simulink model "Simulacion_2"  (R2021b)
settings: Solver=VariableStepAuto  StartTime=0.0  StopTime=1/60  MaxStep=0.0001  MinStep=0.00001  RelTol=1e-3
libraries: spsSeriesRLCBranchLib x6, spsACVoltageSourceLib x3, spsCurrentMeasurementLib x3, spsPowerLib x3, spsVoltageMeasurementLib x3, spsNeutralLib x1, spspowerguiLib x1
settings Model: Creator=Roberto  LastModifiedBy=Roberto

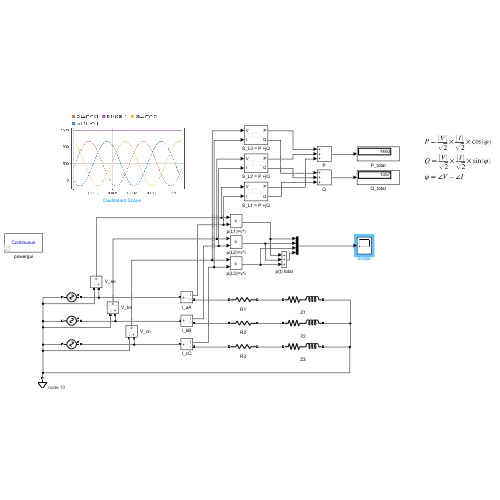
[thumbnail: Simulink's stored preview of the top-level diagram]
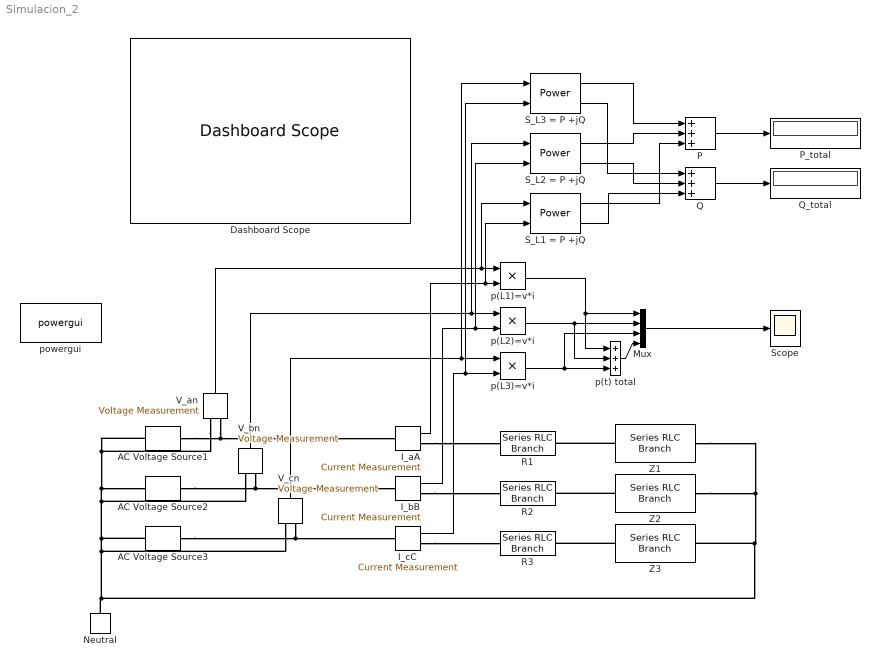
== system Simulacion_2 ==
  AC Voltage Source1 : spsACVoltageSourceLib/AC Voltage Source  Amplitude=100  Phase=0  Frequency=60  SampleTime=0  Measurements=None  BusType=swing  Pref=10e3  Qref=0  Qmin=-inf  Qmax=+inf
  AC Voltage Source2 : spsACVoltageSourceLib/AC Voltage Source  Amplitude=100  Phase=240  Frequency=60  SampleTime=0  Measurements=None  BusType=swing  Pref=10e3  Qref=0  Qmin=-inf  Qmax=+inf
  AC Voltage Source3 : spsACVoltageSourceLib/AC Voltage Source  Amplitude=100  Phase=120  Frequency=60  SampleTime=0  Measurements=None  BusType=swing  Pref=10e3  Qref=0  Qmin=-inf  Qmax=+inf
  Dashboard Scope : DashboardScope
  I_aA : spsCurrentMeasurementLib/Current Measurement  PhasorSimulation=off  OutputType=Complex  PSBequivalent=0
  I_bB : spsCurrentMeasurementLib/Current Measurement  PhasorSimulation=off  OutputType=Complex  PSBequivalent=0
  I_cC : spsCurrentMeasurementLib/Current Measurement  PhasorSimulation=off  OutputType=Complex  PSBequivalent=0
  Mux : Mux
  Neutral : spsNeutralLib/Neutral  LConnTagsString=a  NodeNumber=10
      settings: AttributesFormatString=node %<NodeNumber>  SourceProductBaseCode=PS
  P : Sum  Inputs=+++
  P_total : Display
  Q : Sum  Inputs=+++
  Q_total : Display
  R1 : spsSeriesRLCBranchLib/Series RLC Branch  LConnTagsString=__new0  RConnTagsString=__new0  BranchType=R  Resistance=0.5  Inductance=1e-3  SetiL0=off  InitialCurrent=0  Capacitance=1e-6  Setx0=off  InitialVoltage=0  Measurements=None
  R2 : spsSeriesRLCBranchLib/Series RLC Branch  LConnTagsString=__new0  RConnTagsString=__new0  BranchType=R  Resistance=0.5  Inductance=1e-3  SetiL0=off  InitialCurrent=0  Capacitance=1e-6  Setx0=off  InitialVoltage=0  Measurements=None
  R3 : spsSeriesRLCBranchLib/Series RLC Branch  LConnTagsString=__new0  RConnTagsString=__new0  BranchType=R  Resistance=0.5  Inductance=1e-3  SetiL0=off  InitialCurrent=0  Capacitance=1e-6  Setx0=off  InitialVoltage=0  Measurements=None
  S_L1 = P +jQ : spsPowerLib/Power  Freq=60  Vinit=[1, 0]  Iinit=[1, 0]  Ts=0
      settings: SourceProductBaseCode=PS
  S_L2 = P +jQ : spsPowerLib/Power  Freq=60  Vinit=[1, 0]  Iinit=[1, 0]  Ts=0
      settings: SourceProductBaseCode=PS
  S_L3 = P +jQ : spsPowerLib/Power  Freq=60  Vinit=[1, 0]  Iinit=[1, 0]  Ts=0
      settings: SourceProductBaseCode=PS
  Scope : Scope
  V_an : spsVoltageMeasurementLib/Voltage Measurement  PhasorSimulation=off  OutputType=Complex  PSBequivalent=0
  V_bn : spsVoltageMeasurementLib/Voltage Measurement  PhasorSimulation=off  OutputType=Complex  PSBequivalent=0
  V_cn : spsVoltageMeasurementLib/Voltage Measurement  PhasorSimulation=off  OutputType=Complex  PSBequivalent=0
  Z1 : spsSeriesRLCBranchLib/Series RLC Branch  LConnTagsString=__new0  RConnTagsString=__new0  BranchType=RL  Resistance=5  Inductance=5/(2*pi*60)  SetiL0=off  InitialCurrent=0  Capacitance=1e-6  Setx0=off  InitialVoltage=0  Measurements=None
  Z2 : spsSeriesRLCBranchLib/Series RLC Branch  LConnTagsString=__new0  RConnTagsString=__new0  BranchType=RL  Resistance=5  Inductance=5/(2*pi*60)  SetiL0=off  InitialCurrent=0  Capacitance=1e-6  Setx0=off  InitialVoltage=0  Measurements=None
  Z3 : spsSeriesRLCBranchLib/Series RLC Branch  LConnTagsString=__new0  RConnTagsString=__new0  BranchType=RL  Resistance=5  Inductance=5/(2*pi*60)  SetiL0=off  InitialCurrent=0  Capacitance=1e-6  Setx0=off  InitialVoltage=0  Measurements=None
  p(L1)=v*i : Product
  p(L2)=v*i : Product
  p(L3)=v*i : Product
  p(t) total : Sum  Inputs=+++
  powergui : spspowerguiLib/powergui  Priority=1  SimulationMode=Continuous  SampleTime=50e-6  frequency=60  Iterations=50  frequencyindice=60  Pbase=100e6  ErrMax=1e-4  UnitsV=kV  UnitsW=MW  buscounter=0  FunctionMessages=off  echomessages=off  EnableUseOfTLC=off  CurrentSourceSwitches=off  DisableSnubberDevices=off  DisableRonSwitches=off  DisableVfSwitches=off  DisplayEquations=off  AutomaticDiscreteSolvers=off  SolverType=Tustin/Backward Euler (TBE)  Interpol=off  ExternalGateDelay=off  methode=off  Ts=100  x0status=blocks  SPID=on  SwTol=0  HookPort=off  NonlinearTolerance=1e-4  nMaxIteration=100  ContinueOnMaxIteration=off  RestoreLinks=warning  ResistiveCurrentMeasurement=off  Frange=[0:2:500]  Ylog=off  Xlog=on  ShowGrid=off  save=off  variable=ZData  structure=0  ZoomFFT=off  StartTime=0.0  cycles=1  DisplayStyle=1  fundamental=60  FreqAxis=off  MaxFrequency=1000  frequencyindicesteady=1  RmsSteady=1  display=off
  wires:
  V_cn/1 -> S_L3 = P +jQ/1, p(L3)=v*i/1
  V_bn/1 -> S_L2 = P +jQ/1, p(L2)=v*i/1
  V_an/1 -> S_L1 = P +jQ/1, p(L1)=v*i/1
  I_aA/1 -> S_L1 = P +jQ/2, p(L1)=v*i/2
  I_cC/1 -> S_L3 = P +jQ/2, p(L3)=v*i/2
  p(L2)=v*i/1 -> p(t) total/2, Mux/2
  p(L3)=v*i/1 -> Mux/3, p(t) total/3
  p(t) total/1 -> Mux/4
  p(L1)=v*i/1 -> Mux/1, p(t) total/1
  I_bB/1 -> S_L2 = P +jQ/2, p(L2)=v*i/2
  S_L3 = P +jQ/1 -> P/1
  S_L2 = P +jQ/1 -> P/2
  S_L1 = P +jQ/1 -> P/3
  S_L3 = P +jQ/2 -> Q/1
  S_L2 = P +jQ/2 -> Q/2
  S_L1 = P +jQ/2 -> Q/3
  Q/1 -> Q_total/1
  P/1 -> P_total/1
  Mux/1 -> Scope/1
  connections:
  I_cC/RConn1 -- R3/LConn1
  I_bB/RConn1 -- R2/LConn1
  I_aA/RConn1 -- R1/LConn1
  AC Voltage Source1/RConn1 -- V_an/LConn1 -- I_aA/LConn1
  AC Voltage Source2/RConn1 -- V_bn/LConn1 -- I_bB/LConn1
  AC Voltage Source3/RConn1 -- V_cn/LConn1 -- I_cC/LConn1
  Z1/LConn1 -- R1/RConn1
  Z2/LConn1 -- R2/RConn1
  Z3/LConn1 -- R3/RConn1
  Z1/RConn1 -- Z2/RConn1 -- Neutral/LConn1 -- V_bn/LConn2 -- AC Voltage Source1/LConn1 -- V_an/LConn2 -- AC Voltage Source2/LConn1 -- AC Voltage Source3/LConn1 -- V_cn/LConn2 -- Z3/RConn1
